simulink model "Parallel"  (R2020a)
settings: Solver=VariableStepAuto  StartTime=0.0  StopTime=6594  RelTol=1e-3
values from neighbouring files (symbols this model uses):
  diff_gear = 3.89    [Parallel_script.m]    (also in Series_script.m = 4.533)
  EM_gear_ratio = 4.533    [Parallel_script.m]    (also in Series_script.m = 1)
  gear_down = [2.1238 16.0393 30.2609 60.0625 97.9696]    [Parallel_script.m]    (also in Series_script.m = [])
  gear_eff = 0.95    [Parallel_script.m]    (also in Series_script.m = 0.98)
  gear_idling_loss = 300    [Parallel_script.m]    (also in Series_script.m = 0)
  gear_ratio = [3.6657 2.4933 1.7945 1.3201 0.9386 0.6875]    [Parallel_script.m]    (also in Series_script.m = [1])
  gear_up = [9.6305 35.4860 46.8741 82.1634 170.9009]    [Parallel_script.m]    (also in Series_script.m = [])
  Gears = 6    [Parallel_script.m]    (also in Series_script.m = 1)
  max_CE_power = 100    [Parallel_script.m]    (also in Series_script.m = 60)
  max_EM_power = 84    [Parallel_script.m]    (also in Series_script.m = 90)
  max_SOC = 0.60    (= 0.6)    [Parallel_script.m]    (also in Series_script.m = 0.5)
  min_SOC = 0.35    [Parallel_script.m]    (also in Series_script.m = 0.3)
  Parallel_add_Mass = 150    [Parallel_script.m]
  T_CE_max = p_me_max*V_d/(2*pi*2)    [Parallel_script.m]    (also in Series_script.m)
  T_EM_max = T_EM_max * max_EM_power*1000/max_EM_power_old    [Parallel_script.m]    (also in Series_script.m)
  V_Mass = 1920    [Parallel_script.m]    (also in Series_script.m)
  V_wheel_dia = 0.739    [Parallel_script.m]    (also in Series_script.m)
  w_CE_min = 105    [Parallel_script.m]
undefined symbols (not defined in the file or in its folder): automatic_gearbox, eta_EM_map, H_u, P_aux, P_CE_cutoff, P_CE_idle, r, T_CE_cutoff, theta_CE, theta_EM, V_CE_map, w_CE_idle, w_CE_max, w_CE_upper, w_EM_max, w_EM_row, w_EM_upper
libraries: qss_tb_library x7
settings Model: Creator=Rahul Pai  LastModifiedBy=Rahul Pai

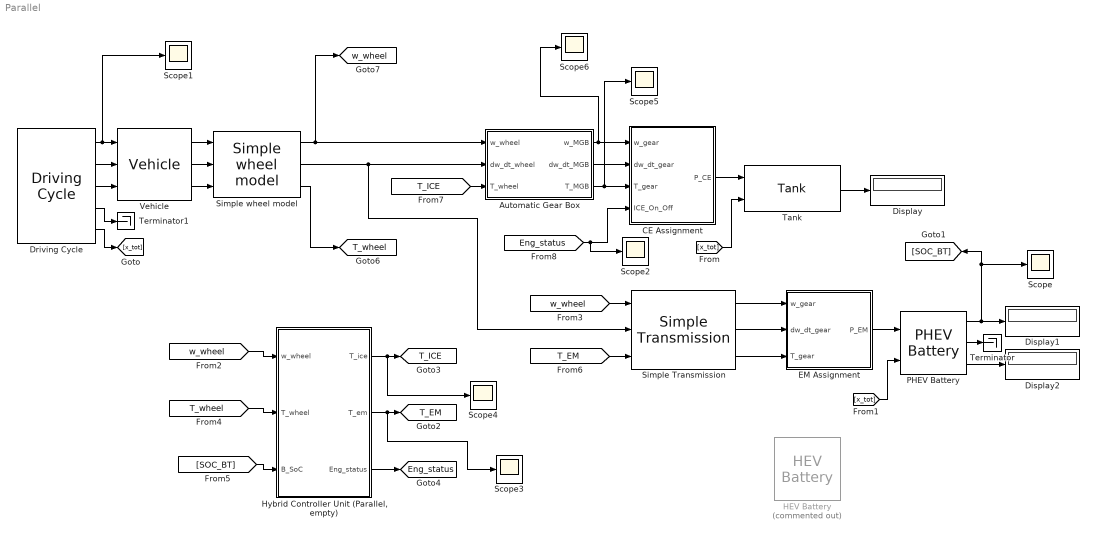
== system Parallel ==
  Automatic Gear Box : Subsystem  Tag=transmission  AncestorBlock=qss_tb_library/Gear System/Automatic Gear Box  mask(Automatic Gear Box){nog=Gears, i=gear_ratio, i_diff=diff_gear, gearon=gear_up, gearoff=gear_down, d=V_wheel_dia, e_GT=gear_eff, P_GT0=gear_idling_loss, w_wheel_min=1}
      mask prompts: nog "Number of gears"; i "Gear ratio vector"; i_diff "Differential gear [-]"; gearon "Switching points for upshift [km/h]"; gearoff "Switching points for downshift [km/h]"; d "Wheel diameter"; e_GT "Efficiency [-]"; P_GT0 "Idling losses (friction) [W]"; w_wheel_min "Minimum wheel speed beyond which losses are generated [rad/s]"
      mask help:
      | This block simulates a automatic gear box, can handle up to 16 gears.
      |
      | Input:
      | =====
      | 	w_wheel	Speed of the wheel [rad/s]
      | 	dw_dt_wheel	Acceleration of the wheel [rad/s^2],
      | 	T_wheel	Torque on the wheel [Nm]
      | 	i	Gear number [-]
      |
      | Output:
      | ======
      | 	w_MGB	Speed of the fly wheel [rad/s]
      | 	dw_dt_MGB	Acceleration of the fly wheel [rad/s^2]
      | 	T_MGB	Torque on the fly wheel [Nm]
      |
      | Number of gears:
      | ======
      | Specify the number of forward gears
      |
      | Shifting points for upshift:
      | ======
      | Vector specifying the velocity for shifting
      | [first_to_second_gear    second_to_third_gear    ....]
      | The number of elements in the vector should be Number of gears - 1.
      |
      | Shifting points for udownshift:
      | ======
      | Simular to upshift
      | [second_to_first_gear    third_to_second_gear    ....]
      mask init:
      | init_AGB;
  CE Assignment : Subsystem  Tag=combustion engine  AncestorBlock=qss_tb_library/Energy Converter/CE Assignment  mask(Combustion Engine (based on consumption map)){engine_type=Gasoline, P_ice=max_CE_power, ENABLE_FUEL_CUTOFF=on}
      mask prompts: engine_type "Engine type"; P_ice "Power [kW]"; ENABLE_FUEL_CUTOFF "Enable fuel cutoff"
      mask help:
      | This block simulates the behaviour of a combustion engine. The block is based on consumption maps for medium sized passenger cars.
      |
      | NA Gasoline:
      | max power @ 5000 rpm
      | max torque @ 3000 rpm
      |
      | Small Diesel:
      | max power @ 4500 rpm
      | max torque @ 2000 rpm
      |
      | Large Diesel:
      | max power @ 1500 rpm
      | max torque @ 1500 rpm
      |
      |
      | Input:
      | =====
      | 	w_gear	Speed of the fly wheel [rad/s]
      | 	dw_dt_gear	Acceleration of the fly wheel [rad/s^2]
      | 	T_gear	Torque on the fly wheel [Nm]
      |
      | Output:
      | ======
      | 	P_CE	Fuel power consumed by the combustion engine [W]
      mask init:
      | init_AssCE_map;
      mask TypeOptions engine_type: Gasoline | Small Diesel | Large Diesel
  Display : Display
  Display1 : Display
  Display2 : Display
  Driving Cycle : qss_tb_library/Driving Cycle/Driving Cycle  Tag=cycle  cyclename1=assignment2_custom_cycle_full  stepsize=1  autostop=on
  EM Assignment : Subsystem  AncestorBlock=qss_tb_library/Energy Converter/EM Assignment  mask(Electric Motor){P_em=max_EM_power}
      mask prompts: P_em "Power [kW]"
      mask help:
      | This block simulates the behaviour of an electric motor. The block is based on an efficiency map. The map is located in the Data/EnergyConvertter/ElectricMotor directory.
      |
      | Maximum speed och the electric motor is 6000 rpm
      | Field weakening region starts at 1500 rpm
      | Maximum mechanical power is at 2150 rpm
      | The maximum torque is 5.98 Nm/kW multiplied with the power you select.
      |
      | Input:
      | =====
      | 	w_gear	Speed of the motor [rad/s]
      | 	dw_dt_gear	Acceleration of the motor [rad/s^2]
      | 	T_gear	Torque of the motor [Nm]
      |
      | Output:
      | ======
      | 	P_EM	Electric Power consumed by the  motor [W]
      mask init:
      | init_EM_ass;
  HEV Battery : qss_tb_library/Energy Buffer/HEV Battery  Tag=battery  Commented=on  cell_series=N_series  cell_parallel=N_parallel  Q_BT_IC_rel=Init_SoC
  "Hybrid Controller Unit (Parallel, empty)" : Subsystem  AncestorBlock=|  mask(Hybrid Controller Unit){}
      | qss_tb_library/Controller/Hybrid Controller Unit 
      | (Parallel, empty)
      mask help: Design your control strategy in this block.
      mask init:
      | init_HCU_parallel;
  PHEV Battery : qss_tb_library/Energy Buffer/PHEV Battery  Tag=battery  cell_series=N_series  cell_parallel=N_parallel  Q_BT_IC_rel=Init_SoC
  Scope{,1..6} (7 alike) : Scope
  Simple Transmission : qss_tb_library/Gear System/Simple Transmission  Tag=simple transmission  gear_ratio=EM_gear_ratio  e_GT=EM_gear_eta  P_GT0=EM_idling_loss  w_wheel_min=1
  Simple wheel model : qss_tb_library/Vehicle/Simple wheel model  Tag=simple transmission  d_wheel=V_wheel_dia
  Tank : qss_tb_library/Energy Source/Tank  Tag=tank  fuel=Gasoline  flag_cold_start=on
  Terminator : Terminator
  Terminator1 : Terminator
  Vehicle : qss_tb_library/Vehicle/Vehicle  Tag=vehicle  m_f=V_Mass+Parallel_add_Mass  A_f=V_area  cw=V_d  mu=V_RRC  k_inertia=V_Rotating
  tag scope: Eng_status=global, T_EM=global, T_ICE=global, T_wheel=global, w_wheel=global
  wires:
  Driving Cycle/1 -> Scope1/1, Vehicle/1
  Driving Cycle/2 -> Vehicle/2
  Driving Cycle/3 -> Vehicle/3
  Vehicle/1 -> Simple wheel model/1
  Vehicle/2 -> Simple wheel model/2
  Vehicle/3 -> Simple wheel model/3
  Tank/1 -> Display/1
  CE Assignment/1(P_CE) -> Tank/1
  EM Assignment/1(P_EM) -> PHEV Battery/1
  Driving Cycle/5 -> [x_tot]
  [x_tot] -> Tank/2
  [x_tot] -> PHEV Battery/2
  PHEV Battery/1 -> [SOC_BT], Scope/1, Display1/1
  PHEV Battery/3 -> Display2/1
  PHEV Battery/2 -> Terminator/1
  Driving Cycle/4 -> Terminator1/1
  Simple Transmission/1 -> EM Assignment/1(w_gear)
  Simple Transmission/2 -> EM Assignment/2(dw_dt_gear)
  Simple Transmission/3 -> EM Assignment/3(T_gear)
  Automatic Gear Box/1(w_MGB) -> Scope6/1, CE Assignment/1(w_gear)
  Automatic Gear Box/2(dw_dt_MGB) -> CE Assignment/2(dw_dt_gear)
  Automatic Gear Box/3(T_MGB) -> Scope5/1, CE Assignment/3(T_gear)
  Simple wheel model/1 -> [w_wheel], Automatic Gear Box/1(w_wheel)
  [w_wheel] -> Simple Transmission/1
  [w_wheel] -> "Hybrid Controller Unit (Parallel, empty)"/1(w_wheel)
  [T_wheel] -> "Hybrid Controller Unit (Parallel, empty)"/2(T_wheel)
  [SOC_BT] -> "Hybrid Controller Unit (Parallel, empty)"/3(B_SoC)
  Simple wheel model/3 -> [T_wheel]
  "Hybrid Controller Unit (Parallel, empty)"/2(T_em) -> Scope3/1, [T_EM]
  [T_EM] -> Simple Transmission/3
  "Hybrid Controller Unit (Parallel, empty)"/1(T_ice) -> Scope4/1, [T_ICE]
  [T_ICE] -> Automatic Gear Box/3(T_wheel)
  "Hybrid Controller Unit (Parallel, empty)"/3(Eng_status) -> [Eng_status]
  [Eng_status] -> Scope2/1, CE Assignment/4(ICE_On_Off)
  Simple wheel model/2 -> Simple Transmission/2, Automatic Gear Box/2(dw_dt_wheel)

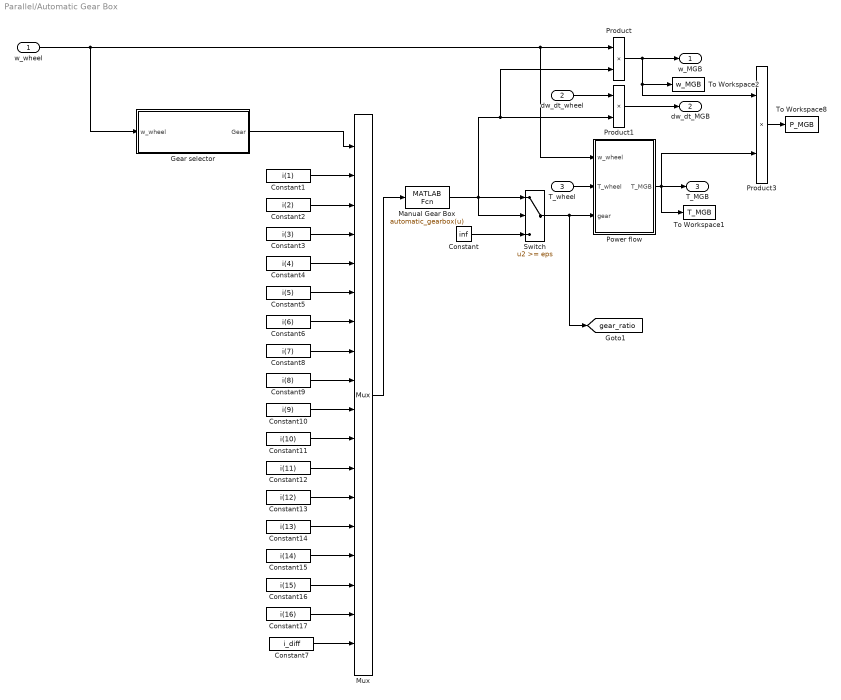
== system Parallel/Automatic Gear Box ==
  w_wheel : Inport
  dw_dt_wheel : Inport  Port=2
  T_wheel : Inport  Port=3
  Constant : Constant  Value=inf
  Constant1 : Constant  Value=i(1)
  Constant10 : Constant  Value=i(9)
  Constant11 : Constant  Value=i(10)
  Constant12 : Constant  Value=i(11)
  Constant13 : Constant  Value=i(12)
  Constant14 : Constant  Value=i(13)
  Constant15 : Constant  Value=i(14)
  Constant16 : Constant  Value=i(15)
  Constant17 : Constant  Value=i(16)
  Constant2 : Constant  Value=i(2)
  Constant3 : Constant  Value=i(3)
  Constant4 : Constant  Value=i(4)
  Constant5 : Constant  Value=i(5)
  Constant6 : Constant  Value=i(6)
  Constant7 : Constant  Value=i_diff
  Constant8 : Constant  Value=i(7)
  Constant9 : Constant  Value=i(8)
  Gear selector : Subsystem
  Manual Gear Box : MATLABFcn  MATLABFcn=automatic_gearbox(u)  OutputDimensions=1
  Mux : Mux  Inputs=18
  Power flow : Subsystem
  Product : Product  InputSameDT=on  RndMeth=Zero  SaturateOnIntegerOverflow=on  OutDataTypeStr=Inherit: Same as first input
  Product1 : Product  InputSameDT=on  RndMeth=Zero  SaturateOnIntegerOverflow=on  OutDataTypeStr=Inherit: Same as first input
  Product3 : Product  InputSameDT=on  RndMeth=Zero  SaturateOnIntegerOverflow=on  OutDataTypeStr=Inherit: Same as first input
  Switch : Switch  Threshold=eps  SaturateOnIntegerOverflow=on  InputSameDT=on
  To Workspace1 : ToWorkspace  VariableName=T_MGB  SampleTime=-1
  To Workspace2 : ToWorkspace  VariableName=w_MGB  SampleTime=-1
  To Workspace8 : ToWorkspace  VariableName=P_MGB  SampleTime=-1
  w_MGB : Outport  InitialOutput=0
  dw_dt_MGB : Outport  Port=2  InitialOutput=0
  T_MGB : Outport  Port=3  InitialOutput=0
  tag scope: gear_ratio=global
  wires:
  Constant17/1 -> Mux/17
  Constant16/1 -> Mux/16
  Constant15/1 -> Mux/15
  Constant14/1 -> Mux/14
  Constant13/1 -> Mux/13
  Constant12/1 -> Mux/12
  Constant11/1 -> Mux/11
  Constant10/1 -> Mux/10
  Constant9/1 -> Mux/9
  Constant8/1 -> Mux/8
  Constant7/1 -> Mux/18
  Power flow/1(T_MGB) -> T_MGB/1, Product3/2, To Workspace1/1
  Product/1 -> w_MGB/1, Product3/1, To Workspace2/1
  Constant/1 -> Switch/3
  w_wheel/1 -> Gear selector/1(w_wheel), Product/1, Power flow/1(w_wheel)
  Product1/1 -> dw_dt_MGB/1
  dw_dt_wheel/1 -> Product1/1
  Manual Gear Box/1 -> Product/2, Product1/2, Switch/2, Switch/1
  Product3/1 -> To Workspace8/1
  Switch/1 -> [gear_ratio], Power flow/3(gear)
  T_wheel/1 -> Power flow/2(T_wheel)
  Constant1/1 -> Mux/2
  Constant2/1 -> Mux/3
  Constant3/1 -> Mux/4
  Constant4/1 -> Mux/5
  Constant5/1 -> Mux/6
  Constant6/1 -> Mux/7
  Gear selector/1(Gear) -> Mux/1
  Mux/1 -> Manual Gear Box/1

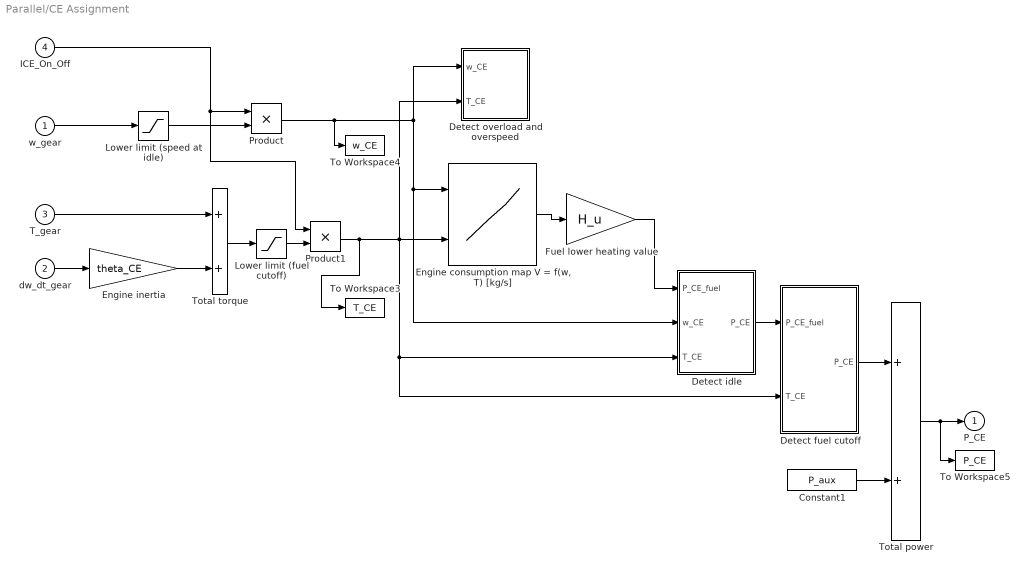
== system Parallel/CE Assignment ==
  w_gear : Inport
  dw_dt_gear : Inport  Port=2
  T_gear : Inport  Port=3
  ICE_On_Off : Inport  Port=4
  Constant1 : Constant  Value=P_aux
  Detect fuel cutoff : Subsystem
  Detect idle : Subsystem
  Detect overload and overspeed : Subsystem
  "Engine consumption map V = f(w, T) [kg/s]" : Lookup2D  RowIndex=w_CE_row  ColumnIndex=T_CE_col  Table=V_CE_map
  Engine inertia : Gain  Gain=theta_CE  SaturateOnIntegerOverflow=on  OutDataTypeStr=Inherit: Same as input  ParamDataTypeStr=Inherit: Same as input
  Fuel lower heating value : Gain  Gain=H_u  SaturateOnIntegerOverflow=on  OutDataTypeStr=Inherit: Same as input  ParamDataTypeStr=Inherit: Same as input
  Lower limit (fuel cutoff) : Saturate  UpperLimit=inf  LowerLimit=T_CE_cutoff
  Lower limit (speed at idle) : Saturate  UpperLimit=inf  LowerLimit=w_CE_idle
  Product : Product
  Product1 : Product
  To Workspace3 : ToWorkspace  VariableName=T_CE  SampleTime=-1
  To Workspace4 : ToWorkspace  VariableName=w_CE  SampleTime=-1
  To Workspace5 : ToWorkspace  VariableName=P_CE  SampleTime=-1
  Total power : Sum  InputSameDT=on  SaturateOnIntegerOverflow=on  OutDataTypeStr=Inherit: Same as first input
  Total torque : Sum  InputSameDT=on  SaturateOnIntegerOverflow=on  OutDataTypeStr=Inherit: Same as first input
  P_CE : Outport  InitialOutput=0
  wires:
  Product1/1 -> To Workspace3/1, Detect fuel cutoff/2(T_CE), Detect idle/3(T_CE), "Engine consumption map V = f(w, T) [kg/s]"/2, Detect overload and overspeed/2(T_CE)
  Constant1/1 -> Total power/2
  Total power/1 -> To Workspace5/1, P_CE/1
  Detect fuel cutoff/1(P_CE) -> Total power/1
  "Engine consumption map V = f(w, T) [kg/s]"/1 -> Fuel lower heating value/1
  Detect idle/1(P_CE) -> Detect fuel cutoff/1(P_CE_fuel)
  Fuel lower heating value/1 -> Detect idle/1(P_CE_fuel)
  w_gear/1 -> Lower limit (speed at idle)/1
  Product/1 -> To Workspace4/1, Detect idle/2(w_CE), "Engine consumption map V = f(w, T) [kg/s]"/1, Detect overload and overspeed/1(w_CE)
  Engine inertia/1 -> Total torque/2
  Total torque/1 -> Lower limit (fuel cutoff)/1
  dw_dt_gear/1 -> Engine inertia/1
  T_gear/1 -> Total torque/1
  Lower limit (speed at idle)/1 -> Product/2
  Lower limit (fuel cutoff)/1 -> Product1/2
  ICE_On_Off/1 -> Product1/1, Product/1

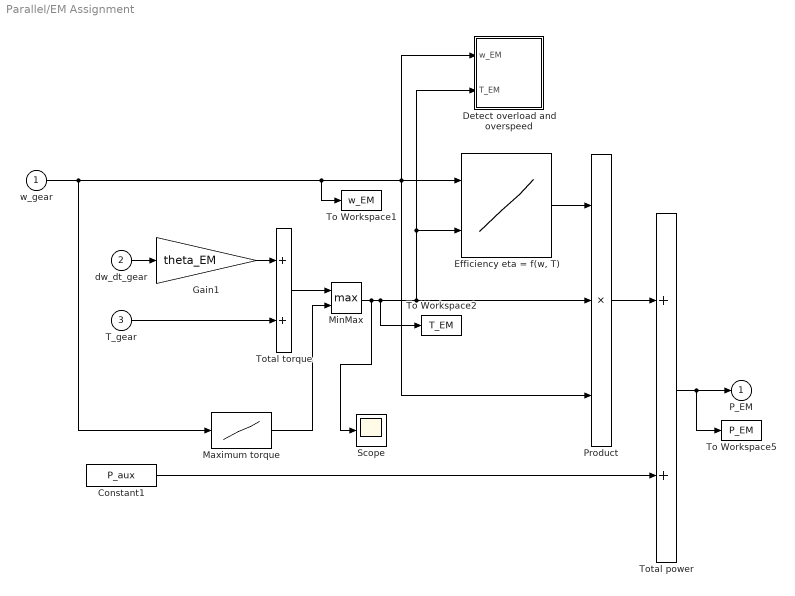
== system Parallel/EM Assignment ==
  w_gear : Inport
  dw_dt_gear : Inport  Port=2
  T_gear : Inport  Port=3
  Constant1 : Constant  Value=P_aux
  Detect overload and overspeed : Subsystem
  "Efficiency eta = f(w, T)" : Lookup2D  RowIndex=w_EM_row  ColumnIndex=T_EM_col  Table=eta_EM_map
  Gain1 : Gain  Gain=theta_EM  SaturateOnIntegerOverflow=on  OutDataTypeStr=Inherit: Same as input  ParamDataTypeStr=Inherit: Same as input
  Maximum torque : Lookup  InputValues=w_EM_row  Table=-T_EM_max  SaturateOnIntegerOverflow=on
  MinMax : MinMax  Function=max  Inputs=2
  Product : Product  Inputs=3  InputSameDT=on  RndMeth=Zero  SaturateOnIntegerOverflow=on  OutDataTypeStr=Inherit: Same as first input
  Scope : Scope
  To Workspace1 : ToWorkspace  VariableName=w_EM  SampleTime=-1
  To Workspace2 : ToWorkspace  VariableName=T_EM  SampleTime=-1
  To Workspace5 : ToWorkspace  VariableName=P_EM  SampleTime=-1
  Total power : Sum  InputSameDT=on  SaturateOnIntegerOverflow=on  OutDataTypeStr=Inherit: Same as first input
  Total torque : Sum  InputSameDT=on  SaturateOnIntegerOverflow=on  OutDataTypeStr=Inherit: Same as first input
  P_EM : Outport  InitialOutput=0
  wires:
  w_gear/1 -> Maximum torque/1, Detect overload and overspeed/1(w_EM), "Efficiency eta = f(w, T)"/1, Product/3, To Workspace1/1
  "Efficiency eta = f(w, T)"/1 -> Product/1
  dw_dt_gear/1 -> Gain1/1
  T_gear/1 -> Total torque/2
  Gain1/1 -> Total torque/1
  MinMax/1 -> Scope/1, To Workspace2/1, Detect overload and overspeed/2(T_EM), "Efficiency eta = f(w, T)"/2, Product/2
  Constant1/1 -> Total power/2
  Product/1 -> Total power/1
  Total power/1 -> P_EM/1, To Workspace5/1
  Total torque/1 -> MinMax/1
  Maximum torque/1 -> MinMax/2

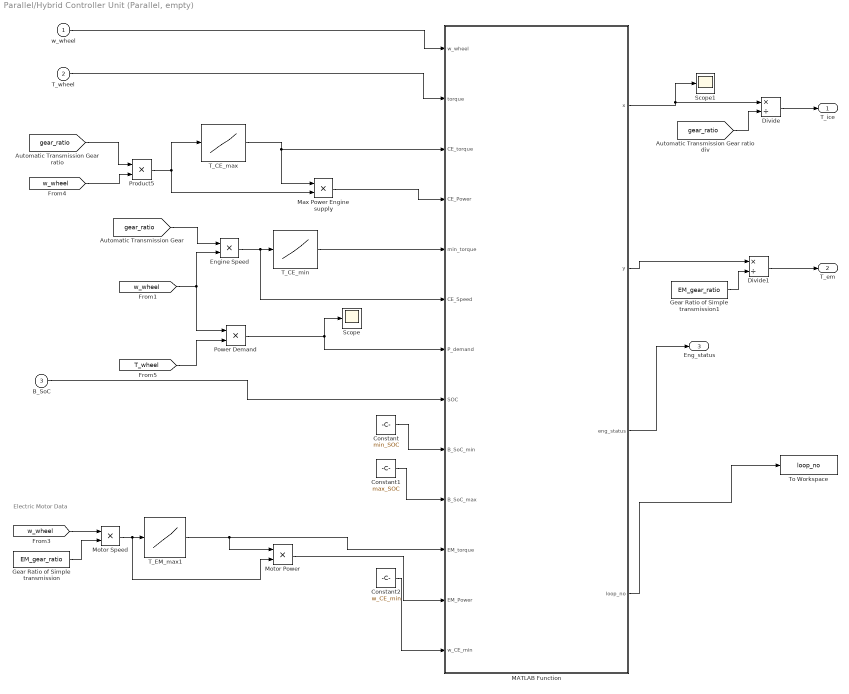
== system Parallel/Hybrid Controller Unit (Parallel, empty) ==
  note: Electric Motor Data
  w_wheel : Inport
  T_wheel : Inport  Port=2
  B_SoC : Inport  Port=3
  Constant : Constant  Value=min_SOC
  Constant1 : Constant  Value=max_SOC
  Constant2 : Constant  Value=w_CE_min
  Divide : Product  Inputs=*/
  Divide1 : Product  Inputs=*/
  Engine Speed : Product
  Gear Ratio of Simple transmission : Constant  Value=EM_gear_ratio
  Gear Ratio of Simple transmission1 : Constant  Value=EM_gear_ratio
  MATLAB Function : MATLAB Function  TreatAsAtomicUnit=on
  Max Power Engine supply : Product
  Motor Power : Product
  Motor Speed : Product
  Power Demand : Product
  Product5 : Product
  Scope : Scope
  Scope1 : Scope
  T_CE_max : Lookup_n-D  NumberOfTableDimensions=1  BreakpointsForDimension1=w_CE_max  Table=T_CE_max  InternalRulePriority=Speed  RndMeth=Simplest  InputSameDT=on
  T_CE_min : Lookup_n-D  NumberOfTableDimensions=1  BreakpointsForDimension1=w_CE_max  Table=0.25*T_CE_max  InternalRulePriority=Speed  RndMeth=Simplest  InputSameDT=on
  T_EM_max1 : Lookup_n-D  NumberOfTableDimensions=1  BreakpointsForDimension1=w_EM_max  Table=T_EM_max  InternalRulePriority=Speed  RndMeth=Simplest  InputSameDT=on
  To Workspace : ToWorkspace  VariableName=loop_no  SaveFormat=Timeseries  SampleTime=-1
  T_ice : Outport  InitialOutput=0
  T_em : Outport  Port=2  InitialOutput=0
  Eng_status : Outport  Port=3  InitialOutput=0
  wires:
  w_wheel/1 -> MATLAB Function/1(w_wheel)
  [gear_ratio] -> Engine Speed/1
  Engine Speed/1 -> MATLAB Function/6(CE_Speed), T_CE_min/1
  T_CE_min/1 -> MATLAB Function/5(min_torque)
  T_wheel/1 -> MATLAB Function/2(torque)
  B_SoC/1 -> MATLAB Function/8(SOC)
  T_EM_max1/1 -> Motor Power/1, MATLAB Function/11(EM_torque)
  Motor Speed/1 -> Motor Power/2, T_EM_max1/1
  Gear Ratio of Simple transmission/1 -> Motor Speed/2
  [w_wheel] -> Motor Speed/1
  Constant/1 -> MATLAB Function/9(B_SoC_min)
  Constant1/1 -> MATLAB Function/10(B_SoC_max)
  Motor Power/1 -> MATLAB Function/12(EM_Power)
  MATLAB Function/2(y) -> Divide1/1
  [w_wheel] -> Power Demand/1, Engine Speed/2
  [T_wheel] -> Power Demand/2
  Power Demand/1 -> Scope/1, MATLAB Function/7(P_demand)
  Product5/1 -> Max Power Engine supply/2, T_CE_max/1
  T_CE_max/1 -> Max Power Engine supply/1, MATLAB Function/3(CE_torque)
  [w_wheel] -> Product5/2
  [gear_ratio] -> Product5/1
  Max Power Engine supply/1 -> MATLAB Function/4(CE_Power)
  MATLAB Function/3(eng_status) -> Eng_status/1
  Constant2/1 -> MATLAB Function/13(w_CE_min)
  MATLAB Function/4(loop_no) -> To Workspace/1
  [gear_ratio] -> Divide/2
  Divide/1 -> T_ice/1
  Gear Ratio of Simple transmission1/1 -> Divide1/2
  Divide1/1 -> T_em/1
  MATLAB Function/1(x) -> Scope1/1, Divide/1

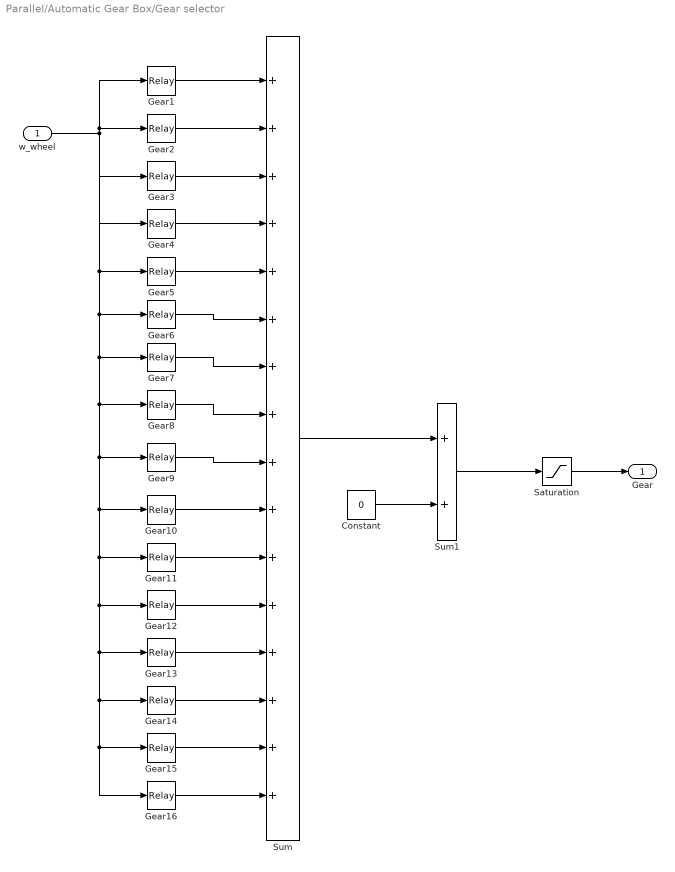
== system Parallel/Automatic Gear Box/Gear selector ==
  w_wheel : Inport
  Constant : Constant  Value=0
  Gear1 : Relay  OffSwitchValue=0
  Gear10 : Relay  OnSwitchValue=gearon(9)/3.6/r  OffSwitchValue=gearoff(9)/3.6/r
  Gear11 : Relay  OnSwitchValue=gearon(10)/3.6/r  OffSwitchValue=gearoff(10)/3.6/r
  Gear12 : Relay  OnSwitchValue=gearon(11)/3.6/r  OffSwitchValue=gearoff(11)/3.6/r
  Gear13 : Relay  OnSwitchValue=gearon(12)/3.6/r  OffSwitchValue=gearoff(12)/3.6/r
  Gear14 : Relay  OnSwitchValue=gearon(13)/3.6/r  OffSwitchValue=gearoff(13)/3.6/r
  Gear15 : Relay  OnSwitchValue=gearon(14)/3.6/r  OffSwitchValue=gearoff(14)/3.6/r
  Gear16 : Relay  OnSwitchValue=gearon(15)/3.6/r  OffSwitchValue=gearoff(15)/3.6/r
  Gear2 : Relay  OnSwitchValue=gearon(1)/3.6/r  OffSwitchValue=gearoff(1)/3.6/r
  Gear3 : Relay  OnSwitchValue=gearon(2)/3.6/r  OffSwitchValue=gearoff(2)/3.6/r
  Gear4 : Relay  OnSwitchValue=gearon(3)/3.6/r  OffSwitchValue=gearoff(3)/3.6/r
  Gear5 : Relay  OnSwitchValue=gearon(4)/3.6/r  OffSwitchValue=gearoff(4)/3.6/r
  Gear6 : Relay  OnSwitchValue=gearon(5)/3.6/r  OffSwitchValue=gearoff(5)/3.6/r
  Gear7 : Relay  OnSwitchValue=gearon(6)/3.6/r  OffSwitchValue=gearoff(6)/3.6/r
  Gear8 : Relay  OnSwitchValue=gearon(7)/3.6/r  OffSwitchValue=gearoff(7)/3.6/r
  Gear9 : Relay  OnSwitchValue=gearon(8)/3.6/r  OffSwitchValue=gearoff(8)/3.6/r
  Saturation : Saturate  UpperLimit=nog  LowerLimit=0
  Sum : Sum  Inputs=16  SaturateOnIntegerOverflow=on
  Sum1 : Sum  Inputs=2  SaturateOnIntegerOverflow=on
  Gear : Outport
  wires:
  Saturation/1 -> Gear/1
  Gear6/1 -> Sum/6
  Gear7/1 -> Sum/7
  Gear8/1 -> Sum/8
  Gear9/1 -> Sum/9
  Gear10/1 -> Sum/10
  Gear11/1 -> Sum/11
  Gear12/1 -> Sum/12
  Gear13/1 -> Sum/13
  Gear14/1 -> Sum/14
  Gear15/1 -> Sum/15
  Gear16/1 -> Sum/16
  Gear5/1 -> Sum/5
  w_wheel/1 -> Gear16/1, Gear15/1, Gear14/1, Gear13/1, Gear12/1, Gear11/1, Gear10/1, Gear9/1, Gear8/1, Gear7/1, Gear6/1, Gear5/1, Gear1/1, Gear2/1, Gear3/1, Gear4/1
  Gear1/1 -> Sum/1
  Gear2/1 -> Sum/2
  Gear3/1 -> Sum/3
  Gear4/1 -> Sum/4
  Sum/1 -> Sum1/1
  Sum1/1 -> Saturation/1
  Constant/1 -> Sum1/2

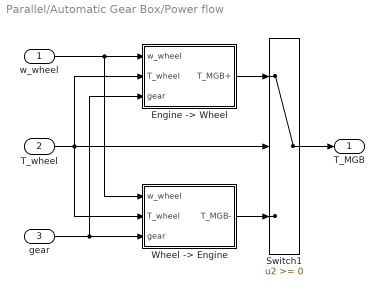
== system Parallel/Automatic Gear Box/Power flow ==
  w_wheel : Inport
  T_wheel : Inport  Port=2
  gear : Inport  Port=3
  "Engine -> Wheel" : Subsystem
  Switch1 : Switch  SaturateOnIntegerOverflow=on  InputSameDT=on
  "Wheel -> Engine" : Subsystem
  T_MGB : Outport  InitialOutput=0
  wires:
  w_wheel/1 -> "Wheel -> Engine"/1(w_wheel), "Engine -> Wheel"/1(w_wheel)
  gear/1 -> "Wheel -> Engine"/3(gear), "Engine -> Wheel"/3(gear)
  "Wheel -> Engine"/1(T_MGB-) -> Switch1/3
  T_wheel/1 -> "Wheel -> Engine"/2(T_wheel), "Engine -> Wheel"/2(T_wheel), Switch1/2
  "Engine -> Wheel"/1(T_MGB+) -> Switch1/1
  Switch1/1 -> T_MGB/1

== system Parallel/CE Assignment/Detect fuel cutoff ==
  P_CE_fuel : Inport
  T_CE : Inport  Port=2
  Constant1 : Constant  Value=ENABLE_FUEL_CUTOFF
  Constant3 : Constant  Value=P_CE_cutoff
  Decision : Switch  Threshold=0.5
  Detect fuel cutoff : Switch  Threshold=T_CE_cutoff + 0.01  SaturateOnIntegerOverflow=on  InputSameDT=on
  P_CE : Outport
  wires:
  Decision/1 -> P_CE/1
  Constant1/1 -> Decision/2
  Detect fuel cutoff/1 -> Decision/1
  P_CE_fuel/1 -> Decision/3, Detect fuel cutoff/1
  T_CE/1 -> Detect fuel cutoff/2
  Constant3/1 -> Detect fuel cutoff/3

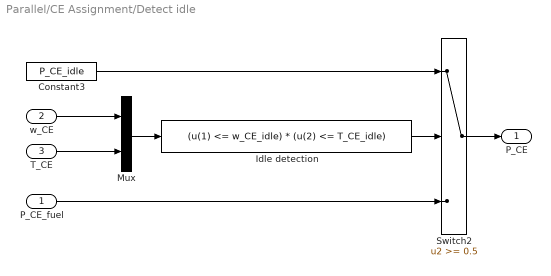
== system Parallel/CE Assignment/Detect idle ==
  P_CE_fuel : Inport
  w_CE : Inport  Port=2
  T_CE : Inport  Port=3
  Constant3 : Constant  Value=P_CE_idle
  Idle detection : Fcn  Expr=(u(1) <= w_CE_idle) * (u(2) <= T_CE_idle)
  Mux : Mux  Inputs=2
  Switch2 : Switch  Threshold=0.5  SaturateOnIntegerOverflow=on  InputSameDT=on
  P_CE : Outport  InitialOutput=0
  wires:
  Constant3/1 -> Switch2/1
  Switch2/1 -> P_CE/1
  P_CE_fuel/1 -> Switch2/3
  Idle detection/1 -> Switch2/2
  w_CE/1 -> Mux/1
  T_CE/1 -> Mux/2
  Mux/1 -> Idle detection/1

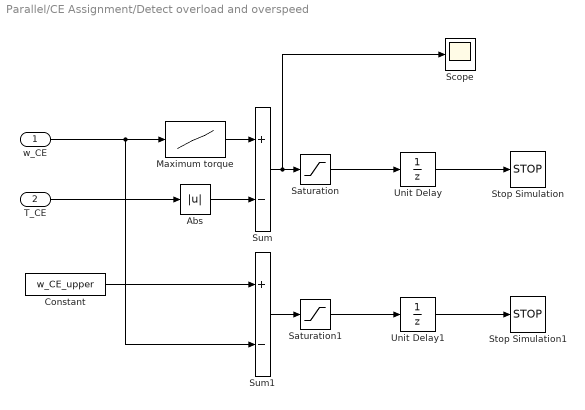
== system Parallel/CE Assignment/Detect overload and overspeed ==
  w_CE : Inport
  T_CE : Inport  Port=2
  Abs : Abs  SaturateOnIntegerOverflow=on
  Constant : Constant  Value=w_CE_upper
  Maximum torque : Lookup  InputValues=w_CE_max  Table=T_CE_max  SaturateOnIntegerOverflow=on
  Saturation : Saturate  UpperLimit=0  LowerLimit=-inf
  Saturation1 : Saturate  UpperLimit=0  LowerLimit=-inf
  Scope : Scope
  Stop Simulation : Stop
  Stop Simulation1 : Stop
  Sum : Sum  Inputs=+-  InputSameDT=on  SaturateOnIntegerOverflow=on  OutDataTypeStr=Inherit: Same as first input
  Sum1 : Sum  Inputs=+-  InputSameDT=on  SaturateOnIntegerOverflow=on  OutDataTypeStr=Inherit: Same as first input
  Unit Delay : UnitDelay  SampleTime=-1  HasFrameUpgradeWarning=on
  Unit Delay1 : UnitDelay  SampleTime=-1  HasFrameUpgradeWarning=on
  wires:
  Unit Delay1/1 -> Stop Simulation1/1
  Unit Delay/1 -> Stop Simulation/1
  Saturation1/1 -> Unit Delay1/1
  Sum1/1 -> Saturation1/1
  Constant/1 -> Sum1/1
  Saturation/1 -> Unit Delay/1
  Abs/1 -> Sum/2
  Maximum torque/1 -> Sum/1
  T_CE/1 -> Abs/1
  w_CE/1 -> Sum1/2, Maximum torque/1
  Sum/1 -> Scope/1, Saturation/1

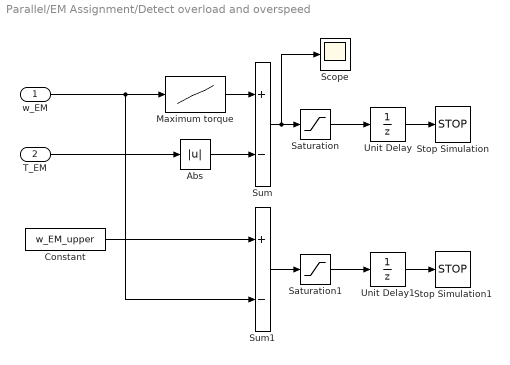
== system Parallel/EM Assignment/Detect overload and overspeed ==
  w_EM : Inport
  T_EM : Inport  Port=2
  Abs : Abs  SaturateOnIntegerOverflow=on
  Constant : Constant  Value=w_EM_upper
  Maximum torque : Lookup  InputValues=w_EM_row  Table=T_EM_max  SaturateOnIntegerOverflow=on
  Saturation : Saturate  UpperLimit=0  LowerLimit=-inf
  Saturation1 : Saturate  UpperLimit=0  LowerLimit=-inf
  Scope : Scope
  Stop Simulation : Stop
  Stop Simulation1 : Stop
  Sum : Sum  Inputs=+-  InputSameDT=on  SaturateOnIntegerOverflow=on  OutDataTypeStr=Inherit: Same as first input
  Sum1 : Sum  Inputs=+-  InputSameDT=on  SaturateOnIntegerOverflow=on  OutDataTypeStr=Inherit: Same as first input
  Unit Delay : UnitDelay  SampleTime=-1  HasFrameUpgradeWarning=on
  Unit Delay1 : UnitDelay  SampleTime=-1  HasFrameUpgradeWarning=on
  wires:
  Unit Delay1/1 -> Stop Simulation1/1
  Unit Delay/1 -> Stop Simulation/1
  Saturation1/1 -> Unit Delay1/1
  Sum1/1 -> Saturation1/1
  Constant/1 -> Sum1/1
  Saturation/1 -> Unit Delay/1
  Abs/1 -> Sum/2
  Maximum torque/1 -> Sum/1
  T_EM/1 -> Abs/1
  w_EM/1 -> Sum1/2, Maximum torque/1
  Sum/1 -> Scope/1, Saturation/1

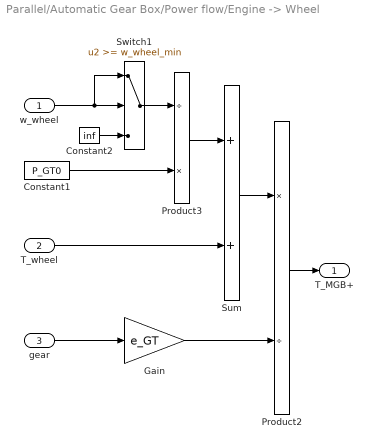
== system Parallel/Automatic Gear Box/Power flow/Engine -> Wheel ==
  w_wheel : Inport
  T_wheel : Inport  Port=2
  gear : Inport  Port=3
  Constant1 : Constant  Value=P_GT0
  Constant2 : Constant  Value=inf
  Gain : Gain  Gain=e_GT  SaturateOnIntegerOverflow=on  OutDataTypeStr=Inherit: Same as input  ParamDataTypeStr=Inherit: Same as input
  Product2 : Product  Inputs=*/  InputSameDT=on  RndMeth=Zero  SaturateOnIntegerOverflow=on  OutDataTypeStr=Inherit: Same as first input
  Product3 : Product  Inputs=/*  InputSameDT=on  RndMeth=Zero  SaturateOnIntegerOverflow=on  OutDataTypeStr=Inherit: Same as first input
  Sum : Sum  InputSameDT=on  SaturateOnIntegerOverflow=on  OutDataTypeStr=Inherit: Same as first input
  Switch1 : Switch  Threshold=w_wheel_min  SaturateOnIntegerOverflow=on  InputSameDT=on
  T_MGB+ : Outport  InitialOutput=0
  wires:
  T_wheel/1 -> Sum/2
  Product3/1 -> Sum/1
  Gain/1 -> Product2/2
  Product2/1 -> T_MGB+/1
  Sum/1 -> Product2/1
  w_wheel/1 -> Switch1/2, Switch1/1
  Constant2/1 -> Switch1/3
  Switch1/1 -> Product3/1
  Constant1/1 -> Product3/2
  gear/1 -> Gain/1

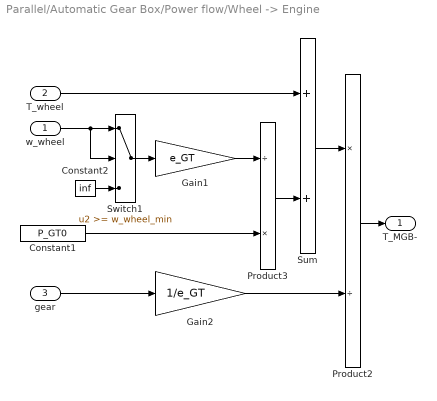
== system Parallel/Automatic Gear Box/Power flow/Wheel -> Engine ==
  w_wheel : Inport
  T_wheel : Inport  Port=2
  gear : Inport  Port=3
  Constant1 : Constant  Value=P_GT0
  Constant2 : Constant  Value=inf
  Gain1 : Gain  Gain=e_GT  SaturateOnIntegerOverflow=on  OutDataTypeStr=Inherit: Same as input  ParamDataTypeStr=Inherit: Same as input
  Gain2 : Gain  Gain=1/e_GT  SaturateOnIntegerOverflow=on  OutDataTypeStr=Inherit: Same as input  ParamDataTypeStr=Inherit: Same as input
  Product2 : Product  Inputs=*/  InputSameDT=on  RndMeth=Zero  SaturateOnIntegerOverflow=on  OutDataTypeStr=Inherit: Same as first input
  Product3 : Product  Inputs=/*  InputSameDT=on  RndMeth=Zero  SaturateOnIntegerOverflow=on  OutDataTypeStr=Inherit: Same as first input
  Sum : Sum  InputSameDT=on  SaturateOnIntegerOverflow=on  OutDataTypeStr=Inherit: Same as first input
  Switch1 : Switch  Threshold=w_wheel_min  SaturateOnIntegerOverflow=on  InputSameDT=on
  T_MGB- : Outport  InitialOutput=0
  wires:
  w_wheel/1 -> Switch1/1, Switch1/2
  gear/1 -> Gain2/1
  Constant2/1 -> Switch1/3
  Switch1/1 -> Gain1/1
  Constant1/1 -> Product3/2
  T_wheel/1 -> Sum/1
  Gain2/1 -> Product2/2
  Product2/1 -> T_MGB-/1
  Product3/1 -> Sum/2
  Sum/1 -> Product2/1
  Gain1/1 -> Product3/1

== matlab function Parallel/Hybrid Controller Unit (Parallel, empty)/MATLAB Function ==
  data: w_wheel input; torque input; CE_torque input; CE_Power input; x output; min_torque input; CE_Speed input; P_demand input; y output; SOC input; B_SoC_min input; B_SoC_max input; EM_torque input; EM_Power input; eng_status output; w_CE_min input; loop_no output
function [x,y,eng_status,loop_no] = fcn(w_wheel,torque,CE_torque,CE_Power,min_torque,CE_Speed,P_demand,SOC,B_SoC_min,B_SoC_max,EM_torque,EM_Power,w_CE_min)
% The power demand is less than zero i.e braking. Then we apply the regenerative braking with the engine off
if P_demand<=0
    y=P_demand/w_wheel;
    x=0;
    eng_status=0;
    loop_no=1;
    % The power demand is greater than zero in this else loop
else
    % If the SoC of the battery is in between then we use the battery in most cases
    if SOC>=B_SoC_min && SOC<B_SoC_max
        % When the speed is below engine speed then motor is run
        if CE_Speed<w_CE_min && P_demand<EM_Power
            x=0;
            y=P_demand/w_wheel;
            eng_status=0;
            loop_no=2;
        end
        % A min torque = 25% of max torque is set where engine is off
        % unless the power demand cannot be met with a motor
        if torque<min_torque && P_demand<=EM_Power
            x=0;
            y=P_demand/w_wheel;
            eng_status=0;
            loop_no=3;
        elseif torque<min_torque && P_demand>EM_Power
            y=EM_torque;
            x=(P_demand-EM_Power)/w_wheel;
            eng_status=1;
            loop_no=4;
            % All other cases with SoC in between
        elseif P_demand<=EM_Power
            x=0;
            y=P_demand/w_wheel;
            eng_status=0;
            loop_no=5;
        else
            y=EM_torque;
            x=(P_demand-EM_Power)/w_wheel;
            eng_status=1;
            loop_no=6;
        end
        % If SoC falls below the minimum
    elseif SOC<B_SoC_min
        % If the power demand is within the engine limits use only engine
        if P_demand<CE_Power
            % If the engine can provide all the torque that the motor can regenerate
            if CE_Power-P_demand>=EM_Power
                y=-EM_torque;
                x=(P_demand+EM_Power)/w_wheel;
                eng_status=1;
                loop_no=7;
            else
                y=-(CE_Power-P_demand)/w_wheel;
                x=CE_torque;
                eng_status=1;
                loop_no=8;
            end
            % If power demand is higher than the engine limit then run the motor
        else
            x=CE_torque;
            y=((P_demand-CE_Power)/w_wheel);
            eng_status=1;
            loop_no=9;
        end
    else
        if P_demand<=EM_Power
            x=0;
            y=P_demand/w_wheel;
            eng_status=0;
            loop_no=10;
        else
            y=EM_torque;
            x=(P_demand-EM_Power)/w_wheel;
            eng_status=1;
            loop_no=11;
        end
    end
end
